simulink model "model_wrapper"  (R2024a)
settings: Solver=VariableStepAuto  StartTime=0.0  StopTime=10.0  RelTol=1e-3
libraries: Crazyflie_Library x1
settings Model: Creator=tinnovosel  LastModifiedBy=tinnovosel

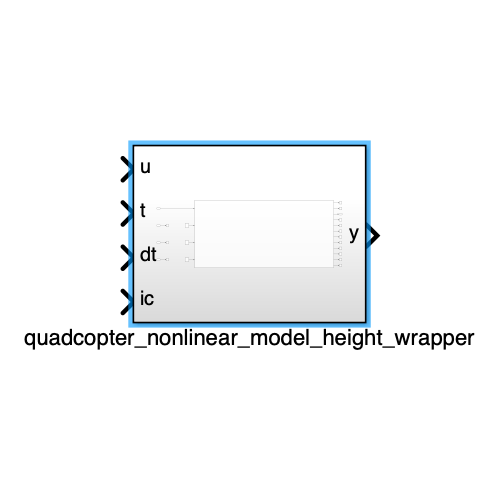
[thumbnail: Simulink's stored preview of the top-level diagram]
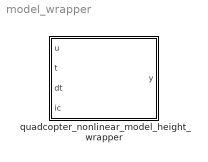
== system model_wrapper ==
  quadcopter_nonlinear_model_height_wrapper : Subsystem

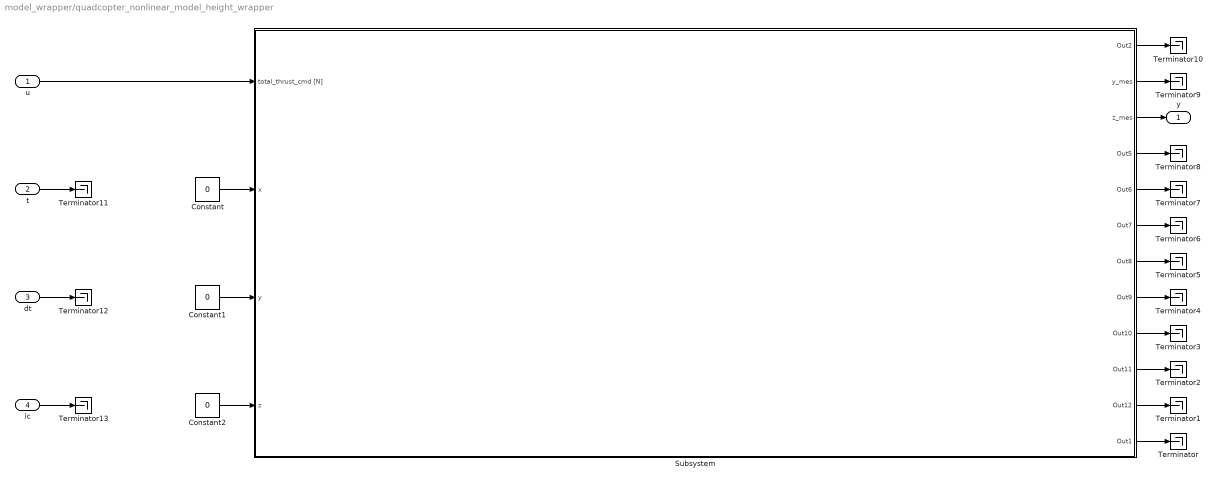
== system model_wrapper/quadcopter_nonlinear_model_height_wrapper ==
  u : Inport  PortDimensions=1
  t : Inport  Port=2
  dt : Inport  Port=3
  ic : Inport  Port=4
  Constant : Constant  Value=0
  Constant1 : Constant  Value=0
  Constant2 : Constant  Value=0
  Subsystem : Subsystem
  Terminator{,1..13} (14 alike) : Terminator
  y : Outport  PortDimensions=1
  wires:
  Subsystem/8(Out9) -> Terminator4/1
  Subsystem/6(Out7) -> Terminator6/1
  Subsystem/1(Out2) -> Terminator10/1
  Subsystem/2(y_mes) -> Terminator9/1
  Subsystem/11(Out12) -> Terminator1/1
  Subsystem/3(z_mes) -> y/1
  Subsystem/5(Out6) -> Terminator7/1
  Subsystem/9(Out10) -> Terminator3/1
  Subsystem/7(Out8) -> Terminator5/1
  Subsystem/10(Out11) -> Terminator2/1
  Subsystem/12(Out1) -> Terminator/1
  Subsystem/4(Out5) -> Terminator8/1
  u/1 -> Subsystem/1(total_thrust_cmd [N])
  Constant/1 -> Subsystem/2(x)
  Constant2/1 -> Subsystem/4(z)
  Constant1/1 -> Subsystem/3(y)
  t/1 -> Terminator11/1
  dt/1 -> Terminator12/1
  ic/1 -> Terminator13/1

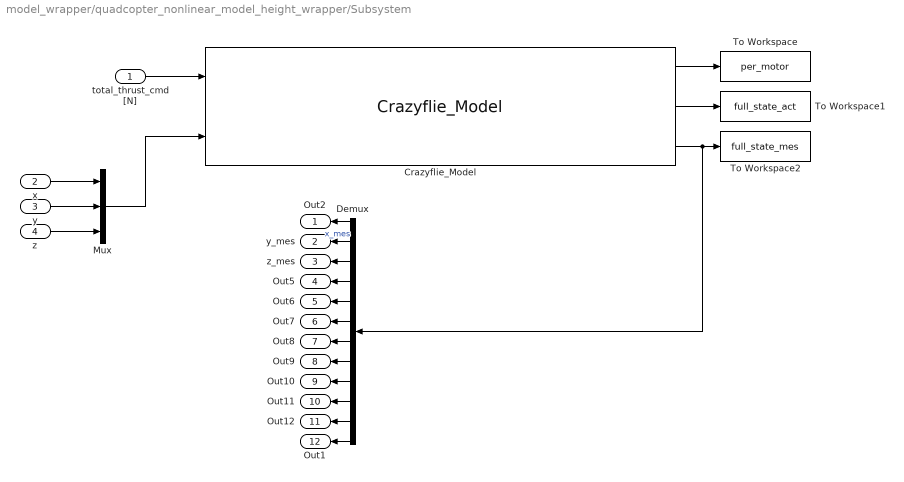
== system model_wrapper/quadcopter_nonlinear_model_height_wrapper/Subsystem ==
  total_thrust_cmd [N] : Inport
  x : Inport  Port=2
  y : Inport  Port=3
  z : Inport  Port=4
  Crazyflie_Model : Crazyflie_Library/Crazyflie_Model  SystemSampleTime=-1  VariantActivationTime=update diagram  AllowFlexibleInterface=on  Latency=0  AutoFrameSizeCalculation=off
  Demux : Demux  Outputs=12
  Mux : Mux  Inputs=3
  To Workspace : ToWorkspace  VariableName=per_motor  SaveFormat=Timeseries  SampleTime=-1
  To Workspace1 : ToWorkspace  VariableName=full_state_act  SaveFormat=Timeseries  SampleTime=-1
  To Workspace2 : ToWorkspace  VariableName=full_state_mes  SaveFormat=Timeseries  SampleTime=-1
  Out2 : Outport
  y_mes : Outport  Port=2
  z_mes : Outport  Port=3
  Out5 : Outport  Port=4
  Out6 : Outport  Port=5
  Out7 : Outport  Port=6
  Out8 : Outport  Port=7
  Out9 : Outport  Port=8
  Out10 : Outport  Port=9
  Out11 : Outport  Port=10
  Out12 : Outport  Port=11
  Out1 : Outport  Port=12
  wires:
  Demux/2 -> y_mes/1  "x_mes"
  total_thrust_cmd [N]/1 -> Crazyflie_Model/1
  Crazyflie_Model/1 -> To Workspace/1
  Crazyflie_Model/3 -> Demux/1, To Workspace2/1
  y/1 -> Mux/2
  Demux/1 -> Out2/1
  x/1 -> Mux/1
  z/1 -> Mux/3
  Mux/1 -> Crazyflie_Model/2
  Crazyflie_Model/2 -> To Workspace1/1
  Demux/3 -> z_mes/1
  Demux/4 -> Out5/1
  Demux/5 -> Out6/1
  Demux/6 -> Out7/1
  Demux/7 -> Out8/1
  Demux/8 -> Out9/1
  Demux/9 -> Out10/1
  Demux/10 -> Out11/1
  Demux/11 -> Out12/1
  Demux/12 -> Out1/1
